simulink library "LeafEcoTronDBWLib"  (R2018a)
settings: Solver=VariableStepAuto  StartTime=0.0  StopTime=10.0  RelTol=1e-3
libraries: Simulink x17, CoderSF_BSW_Libs x3
(part 2 of 2)

== stateflow chart LeafEcoTronDBWLib/SystemStatechart_Arbitration ==
  state Initializing
    entry:
    state = SystemState.INITIALIZING;
    engaged = false;
    selectedSubsystems = MADC_subsystemSelect;
    driverOverridden = false;
    driverOverrideCulprit = uint8(0);
    faultOverridden = false;
    faultOverrideCulprit = uint8(0);
    faultOverrideCounter = uint8(0);
    driverOverrideCounter = uint8(0);
    waitingForDriverActivity = false;
    waitingForOverrideClear = false;
    buzzer = false;
    arbitratorState = ArbitratorState.HUMAN;
    state LedsOff
      entry:
      redLED = LEDState.LED_OFF;
      yellowLED = LEDState.LED_OFF;
      greenLED = LEDState.LED_OFF;
    state RedLedOn
      entry:
      redLED = LEDState.LED_ON;
      yellowLED = LEDState.LED_OFF;
      greenLED = LEDState.LED_OFF;
    state YellowLedOn
      entry:
      redLED = LEDState.LED_OFF;
      yellowLED = LEDState.LED_ON;
      greenLED = LEDState.LED_OFF;
    state GreenLedOn
      entry:
      redLED = LEDState.LED_OFF;
      yellowLED = LEDState.LED_OFF;
      greenLED = LEDState.LED_ON;
    state AllLedsOn
      entry:
      redLED = LEDState.LED_ON;
      yellowLED = LEDState.LED_ON;
      greenLED = LEDState.LED_ON;
    (default) -> LedsOff
    LedsOff -> RedLedOn : after(1000, tick)
    RedLedOn -> YellowLedOn : after(1000, tick)
    YellowLedOn -> GreenLedOn : after(1000, tick)
    GreenLedOn -> AllLedsOn : after(1000, tick)
  state ADSDisengaged
    state PreOperational
      entry:
      arbitratorState = ArbitratorState.HUMAN;
      driverOverrideCulprit = uint8(0); faultOverrideCulprit = uint8(0);
      during: selectedSubsystems = MADC_subsystemSelect;
      state LLC [parallel]
        settings: executionOrder=1
        state LLCNotReady
          entry:
          state = SystemState.NOT_READY;
          redLED = LEDState.LED_ON;
          yellowLED = LEDState.LED_OFF;
        state LLCReady
          entry:
          state = SystemState.READY;
          redLED = LEDState.LED_OFF;
          yellowLED = LEDState.LED_ON;
        (default) -> LLCNotReady
        LLCReady -> LLCNotReady : [vehicleFault]
        LLCNotReady -> LLCReady : [~vehicleFault]
      state ADC [parallel]
        settings: executionOrder=2
        state ADCNotReady
          entry:
          greenLED = LEDState.LED_OFF;
        state ADCReady
          entry:
          greenLED = LEDState.LED_SLOW_PULSE;
        (default) -> ADCNotReady
        ADCReady -> ADCNotReady : [~(MADC_capable || ...
            |      RADC_capable)]
        ADCNotReady -> ADCReady : [MADC_capable && RADC_capable]
    state FaultOverridden
      entry:
      state = SystemState.FAULT_OVERRIDDEN;
      arbitratorState = ArbitratorState.EMERGENCY_AEB;
      engaged = false;
      faultOverridden = true;
      exit:
      faultOverridden = false;
      state WaitingForADC
        entry:
        waitingForOverrideClear = true;
        redLED = LEDState.LED_ON;
        yellowLED = LEDState.LED_OFF;
        greenLED = LEDState.LED_OFF;
        exit:
        waitingForOverrideClear = false;
      state AlertingDriver
        entry:
        buzzer = true;
        redLED = LEDState.LED_FAST_PULSE;
        yellowLED = LEDState.LED_FAST_PULSE;
        greenLED = LEDState.LED_FAST_PULSE;
      state WaitingForDriverActivity
        entry:
        waitingForDriverActivity = true;
        exit:
        buzzer = false;
        waitingForDriverActivity = false;
      ADSDisengaged.FaultOverridden.AlertingDriver -> ADSDisengaged.FaultOverridden.WaitingForDriverActivity : after(500,tick)
      ADSDisengaged.FaultOverridden.WaitingForDriverActivity -> ADSDisengaged.FaultOverridden.WaitingForADC : [driverActivity || selectedSubsystems == 1 || selectedSubsystems == 4 || selectedSubsystems == 5]
    state WaitingForDriverActivity
      entry:
      waitingForDriverActivity = true;
      exit:
      buzzer = false;
      waitingForDriverActivity = false;
    state DriverOverridden
      entry:
      state = SystemState.DRIVER_OVERRIDDEN;
      arbitratorState = ArbitratorState.HUMAN;
      engaged = false;
      driverOverridden = true;
      exit:
      driverOverridden = false;
      state AlertingDriver
        entry:
        buzzer = true;
        redLED = LEDState.LED_FAST_PULSE;
        yellowLED = LEDState.LED_FAST_PULSE;
        greenLED = LEDState.LED_FAST_PULSE;
        exit:
        buzzer = false;
      state WaitingForADC
        entry:
        waitingForOverrideClear = true;
        redLED = LEDState.LED_ON;
        yellowLED = LEDState.LED_OFF;
        greenLED = LEDState.LED_OFF;
        exit:
        waitingForOverrideClear = false;
      ADSDisengaged.DriverOverridden.AlertingDriver -> ADSDisengaged.DriverOverridden.WaitingForADC : after(500,tick)
    state ADSRelinquishWarning
      entry:
      state = SystemState.ADS_RELINQUISH_WARNING;
      arbitratorState = ArbitratorState.HUMAN;
      engaged = false;
      buzzer = true;
      redLED = LEDState.LED_FAST_PULSE;
      yellowLED = LEDState.LED_FAST_PULSE;
      greenLED = LEDState.LED_FAST_PULSE;
    ADSDisengaged.DriverOverridden.WaitingForADC -> PreOperational : [(MADC_clearOverride && ~MADC_requestADSEngaged)...
        |   || (RADC_clearOverride && ~RADC_requestADSEngaged)]
    ADSDisengaged.FaultOverridden.WaitingForADC -> PreOperational : [(MADC_clearOverride && ~MADC_requestADSEngaged)...
        |   || (RADC_clearOverride && ~RADC_requestADSEngaged)]
    ADSDisengaged.WaitingForDriverActivity -> PreOperational : [driverActivity || selectedSubsystems == 1 || selectedSubsystems == 4 || selectedSubsystems == 5]
    ADSRelinquishWarning -> ADSDisengaged.WaitingForDriverActivity : after(500,tick)
  state ADSEngaged
    entry:
    engaged = true;
    exit:
    driverOverrideCulprit = driverOverrideByte;
    faultOverrideCulprit = faultOverrideByte;
    state Pending2RADC
      entry:
      state = SystemState.RADC_TRANSFER_PENDING;
    state MADC_Control
      entry:
      state = SystemState.MADC_ENGAGED;
      redLED = LEDState.LED_OFF;
      yellowLED = LEDState.LED_OFF;
      greenLED = LEDState.LED_ON;
    state RADC_WaitForConfirm
      entry:
      state=SystemState.RADC_WAIT_CONFIRM;
      arbitratorState = ArbitratorState.RADC;
      selectedSubsystems = RADC_subsystemSelect;
    state pendingTimeout
    state RADC_Control
      entry:
      state = SystemState.RADC_ENGAGED;
      redLED = LEDState.LED_OFF;
      yellowLED = LEDState.LED_OFF;
      greenLED = LEDState.LED_SLOW_PULSE;
    state MADC_WaitForConfirm
      entry:
      state=SystemState.MADC_WAIT_CONFIRM;
      arbitratorState = ArbitratorState.MADC;
      selectedSubsystems = MADC_subsystemSelect;
    state Pending2MADC
      entry:
      state = SystemState.MADC_TRANSFER_PENDING;
    RADC_WaitForConfirm -> pendingTimeout [order 2] : after(500,tick)
    Pending2RADC -> pendingTimeout [order 1] : after(500, tick)
    MADC_Control -> Pending2RADC [order 1] : [(~MADC_capable) || ...
        | MADC_canFault]
    Pending2RADC -> RADC_WaitForConfirm [order 2] : [[ARB_ctrl2RADC]]
    MADC_Control -> RADC_WaitForConfirm [order 2] : [ARB_ctrl2RADCDirect]
    RADC_WaitForConfirm -> RADC_Control [order 1] : [ARB_RADCInCtrl]
    MADC_WaitForConfirm -> MADC_Control [order 2] : [ARB_MADCInCtrl]
    MADC_WaitForConfirm -> pendingTimeout [order 1] : after(500,tick)
    Pending2MADC -> pendingTimeout [order 2] : after(500,tick)
    (default) -> MADC_WaitForConfirm
    RADC_Control -> MADC_WaitForConfirm [order 2] : [ARB_ctrl2MADC && vehicleStopped]
    Pending2MADC -> MADC_WaitForConfirm [order 1] : [ARB_ctrl2MADC]
    RADC_Control -> Pending2MADC [order 1] : [~RADC_capable || ...
        |  RADC_canFault]
  (default) -> Initializing
  AllLedsOn -> PreOperational : after(1000, tick)
  PreOperational -> ADSEngaged : [~(vehicleFault || MADC_canFault || RADC_canFault) && ...
      |   MADC_capable && MADC_requestADSEngaged && ...
      |   RADC_capable && RADC_requestADSEngaged && ...
      |   (MADC_subsystemSelect ~= 0) && ...
      |   (MADC_subsystemSelect == RADC_subsystemSelect)]
  pendingTimeout -> ADSDisengaged.FaultOverridden.AlertingDriver
  ADSEngaged -> ADSDisengaged.FaultOverridden.AlertingDriver [order 2] : [vehicleFault || (MADC_canFault && RADC_canFault) ||...
      |  ~(MADC_capable || RADC_capable)] ...
      | {faultOverrideCounter = faultOverrideCounter + 1;}
  ADSEngaged -> ADSDisengaged.DriverOverridden.AlertingDriver [order 3] : [driverOverride]{driverOverrideCounter = driverOverrideCounter + 1;}
  ADSEngaged -> ADSRelinquishWarning [order 1] : [(~MADC_requestADSEngaged && arbitratorState == ArbitratorState.MADC) ...
      |  || (~RADC_requestADSEngaged && arbitratorState == ArbitratorState.RADC)]
  data: selectedSubsystems output uint8; engaged output boolean; driverOverridden output boolean; driverOverrideCulprit output uint8; faultOverridden output boolean; faultOverrideCulprit output uint8; waitingForDriverActivity output boolean; waitingForOverrideClear output boolean; faultOverrideCounter output uint8; driverOverrideCounter output uint8; MADC_requestADSEngaged input boolean; RADC_requestADSEngaged input boolean; MADC_subsystemSelect input uint8; RADC_subsystemSelect input uint8; MADC_clearOverride input boolean; RADC_clearOverride input boolean; buzzer output boolean; driverActivity input boolean; driverOverride input boolean; driverOverrideByte input uint8; vehicleFault input boolean; MADC_canFault input boolean; RADC_canFault input boolean; faultOverrideByte input uint8; MADC_capable input boolean; redLED output; yellowLED output; greenLED output; state output; arbitratorState output; RADC_capable input boolean; ARB_ctrl2MADC input; ARB_ctrl2RADC input; ARB_ctrl2RADCDirect input; ARB_MADCInCtrl input; ARB_RADCInCtrl input; vehicleStopped input boolean; remoteControlBrake input boolean

== stateflow chart LeafEcoTronDBWLib/EPBStateChart ==
  state Home
    entry:
    signal1 = false;
    signal2 = false;
    state Wait
    state Ready
    (default) -> Wait
    Wait -> Ready : after(1250, tick)
  state Shifting
  (default) -> Home
  (junction 17) -> Shifting : after(2000, tick)
  (junction 15) -> (junction 17) [order 2] : [commandedEPB == EPBCommand.EPB_RELEASE || SR_unlock == true]
      | {signal1 = false; signal2 = true;}
  Ready -> (junction 15) : [commandedEPB ~= EPBCommand.EPB_NO_ACTION || SR_unlock == true || SR_lock == true]
  (junction 15) -> (junction 16) [order 1] : [commandedEPB == EPBCommand.EPB_APPLY || SR_lock == true]
      | {signal1 = true; signal2 = false;}
  Shifting -> Home : after(1000, tick)
  (junction 16) -> Shifting : after(1000, tick)
  data: signal1 output boolean; signal2 output boolean; commandedEPB input Enum: EPBCommand; vehicleSpeed input single; SR_lock input boolean; SR_unlock input boolean
